simulink model "TTankModel"  (R2017b)
settings: Solver=FixedStepAuto  StartTime=62407  StopTime=120960  FixedStep=0.1  RelTol=1e-3
values from neighbouring files (symbols this model uses):
  intDelay = 20    [SingleFault.m]
  outTr = TTankModel_PCAtrainFunc(Xu_train)    [SingleFault.m]    (also in TTankModel_PCAtrainFunc.m = struct('mu_u',mu_u, 'sig_u',sigma_u,'PA', PA, 'LA', LA, 'A',)
  sizeStep_Gc11 = sensBias(1)    [SingleFault.m]    (also in faultCond.m = 0; steadyStateSet.m = 0)
  sizeStep_Gc23 = sensBias(2)    [SingleFault.m]    (also in faultCond.m = 0; steadyStateSet.m = 0)
  sizeStep_Gc32 = sensBias(3)    [SingleFault.m]    (also in faultCond.m = 0; steadyStateSet.m = 0)
  sizeStep_Gc44 = sensBias(4)    [SingleFault.m]    (also in faultCond.m = sensStep; steadyStateSet.m = 0)
  smDelay = 6    [SingleFault.m]
  tStep_Gc11 = sensTot(1,2)    [SingleFault.m]    (also in faultCond.m = 0; steadyStateSet.m = 0)
  tStep_Gc23 = sensTot(2,2)    [SingleFault.m]    (also in faultCond.m = 0; steadyStateSet.m = 0)
  tStep_Gc32 = sensTot(3,2)    [SingleFault.m]    (also in faultCond.m = 0; steadyStateSet.m = 0)
  tStep_Gc44 = sensTot(4,2)    [SingleFault.m]    (also in faultCond.m = sensTime; steadyStateSet.m = 0)
undefined symbols (not defined in the file or in its folder): ssOut
libraries: simulink x36
settings Model: Creator=17496594  LastModifiedBy=jtmccoy
settings DataIOCC: FinalStateName=SimStateTest  InitialState=stdyState  SaveCompleteFinalSimState=on  SaveFormat=Array  SignalLogging=off
settings CodeAppCC: StateflowObjectComments=on

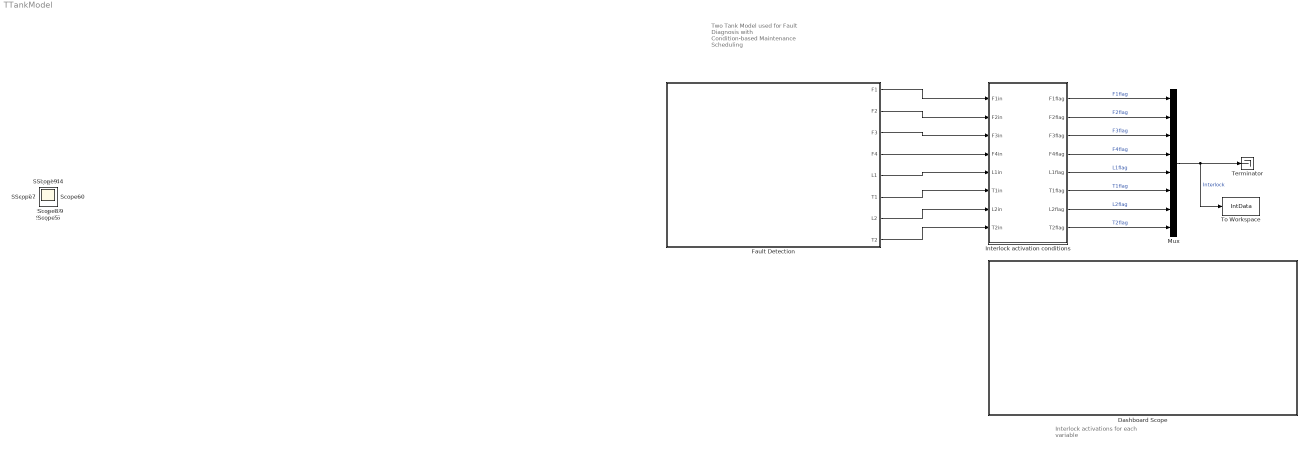
== system TTankModel ==
  note: Two Tank Model used for Fault Diagnosis
      | with Condition-based Maintenance Scheduling
  note: Interlock activations for each variable
  Dashboard Scope : Subsystem  DialogController=hmiCreateDDGDialog  IsWebBlock=on  mask(MWDashboardBlock){webBlockId=f2d3fcda-b4ff-4067-adce-a90dbe78b41d, webBlockType=sdiscope, ShowInitialText=on, HMISrcModelName=TTankModel}
      mask prompts: webBlockId "WebBlock Id"; webBlockType "WebBlock Type"; HMISrcModelName "Source Model"
      mask help: SimulinkHMI:dialogs:HMIScopeDialogDesc
      mask Help: helpview([docroot '/mapfiles/simulink.map'], 'hmi_scope')
      mask Display:
      | if strcmp(get_param(bdroot(gcb),'BlockDiagramType'), 'library')
      |     image([(matlabroot) '/toolbox/simulink/hmi/icons/DashboardScope.png']);
      | end
  Fault Detection : Subsystem
  Interlock activation conditions : Subsystem
  Mux : Mux  Inputs=8
  Terminator : Terminator
  To Workspace : ToWorkspace  VariableName=IntData  SampleTime=1
      settings: Save2DSignal=2-D array (concatenate along first dimension)
  Scope{,1..21} (22 alike) : Scope
  wires:
  Interlock activation conditions/2(F2flag) -> Mux/2  "F2flag"
  Fault Detection/8(T2) -> Interlock activation conditions/8(T2in)
  Fault Detection/7(L2) -> Interlock activation conditions/7(L2in)
  Fault Detection/5(L1) -> Interlock activation conditions/5(L1in)
  Fault Detection/6(T1) -> Interlock activation conditions/6(T1in)
  Fault Detection/4(F4) -> Interlock activation conditions/4(F4in)
  Fault Detection/3(F3) -> Interlock activation conditions/3(F3in)
  Fault Detection/2(F2) -> Interlock activation conditions/2("F2in ")
  Fault Detection/1(F1) -> Interlock activation conditions/1(F1in)
  Interlock activation conditions/8(T2flag) -> Mux/8  "T2flag"
  Mux/1 -> To Workspace/1, Terminator/1  "Interlock"
  Interlock activation conditions/7(L2flag) -> Mux/7  "L2flag"
  Interlock activation conditions/6(T1flag) -> Mux/6  "T1flag"
  Interlock activation conditions/5(L1flag) -> Mux/5  "L1flag"
  Interlock activation conditions/4(F4flag) -> Mux/4  "F4flag"
  Interlock activation conditions/1(F1flag) -> Mux/1  "F1flag"
  Interlock activation conditions/3(F3flag) -> Mux/3  "F3flag"

== system TTankModel/Dashboard Scope ==

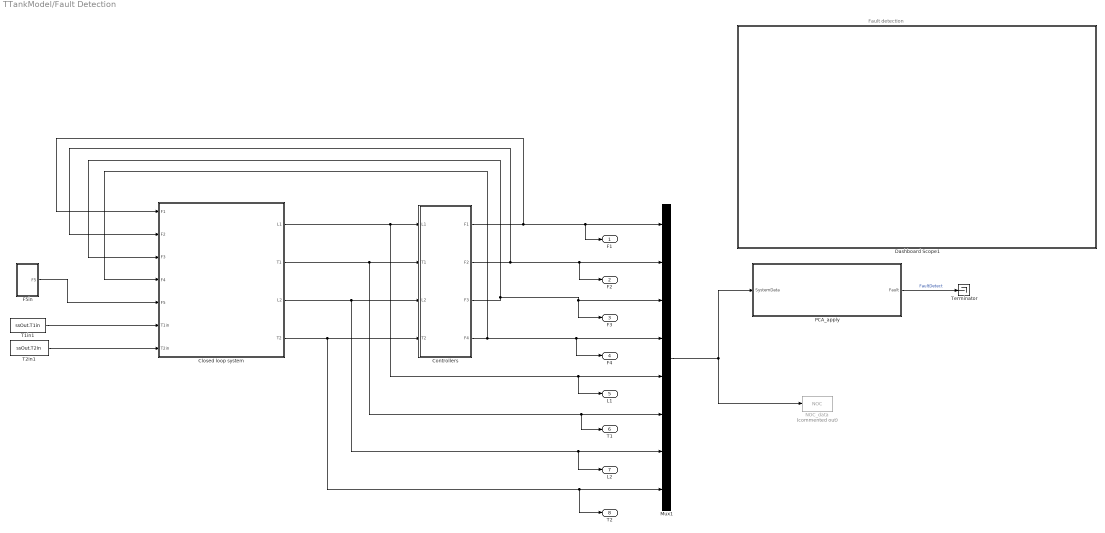
== system TTankModel/Fault Detection ==
  note: Fault detection
  Closed loop system : Subsystem
  Controllers : Subsystem
  Dashboard Scope1 : Subsystem  DialogController=hmiCreateDDGDialog  IsWebBlock=on  mask(MWDashboardBlock){webBlockId=01f67c63-4ebd-45d4-811d-95e04fe09010, webBlockType=sdiscope, ShowInitialText=on, HMISrcModelName=TTankModel}
      mask prompts: webBlockId "WebBlock Id"; webBlockType "WebBlock Type"; HMISrcModelName "Source Model"
      mask help: SimulinkHMI:dialogs:HMIScopeDialogDesc
      mask Help: helpview([docroot '/mapfiles/simulink.map'], 'hmi_scope')
      mask Display:
      | if strcmp(get_param(bdroot(gcb),'BlockDiagramType'), 'library')
      |     image([(matlabroot) '/toolbox/simulink/hmi/icons/DashboardScope.png']);
      | end
  F5in : Subsystem
  Mux1 : Mux  Inputs=8
  NOC_data : ToWorkspace  Commented=on  VariableName=NOC  SaveFormat=Timeseries  SampleTime=1
  PCA_apply : Subsystem
  T1in1 : Constant  Value=ssOut.T1in
  T2in1 : Constant  Value=ssOut.T2in
  Terminator : Terminator
  F1 : Outport
  F2 : Outport  Port=2
  F3 : Outport  Port=3
  F4 : Outport  Port=4
  L1 : Outport  Port=5
  T1 : Outport  Port=6
  L2 : Outport  Port=7
  T2 : Outport  Port=8
  wires:
  PCA_apply/1(Fault) -> Terminator/1  "FaultDetect"
  F5in/1(F5) -> Closed loop system/5(F5)
  Closed loop system/1(L1) -> Controllers/1(L1), L1/1, Mux1/5
  Mux1/1 -> PCA_apply/1(SystemData), NOC_data/1
  T1in1/1 -> Closed loop system/6(T1in)
  T2in1/1 -> Closed loop system/7(T2in)
  Closed loop system/4(T2) -> Controllers/4(T2), T2/1, Mux1/8
  Closed loop system/3(L2) -> Controllers/3(L2), L2/1, Mux1/7
  Closed loop system/2(T1) -> Controllers/2(T1), T1/1, Mux1/6
  Controllers/4(F4) -> Closed loop system/4(F4), F4/1, Mux1/4
  Controllers/2(F2) -> Closed loop system/2(F2), F2/1, Mux1/2
  Controllers/3(F3) -> Closed loop system/3(F3), F3/1, Mux1/3
  Controllers/1(F1) -> Closed loop system/1(F1), F1/1, Mux1/1

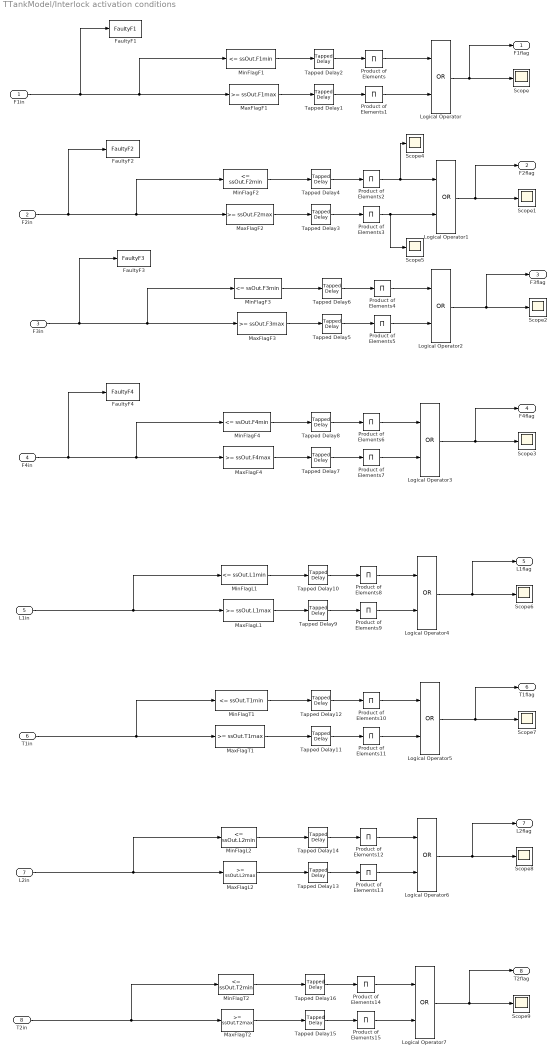
== system TTankModel/Interlock activation conditions ==
  F1in : Inport
  "F2in " : Inport  Port=2
  F3in : Inport  Port=3
  F4in : Inport  Port=4
  L1in : Inport  Port=5
  T1in : Inport  Port=6
  L2in : Inport  Port=7
  T2in : Inport  Port=8
  FaultyF1 : ToWorkspace  VariableName=FaultyF1  SaveFormat=Timeseries  SampleTime=-1
  FaultyF2 : ToWorkspace  VariableName=FaultyF2  SaveFormat=Timeseries  SampleTime=-1
  FaultyF3 : ToWorkspace  VariableName=FaultyF3  SaveFormat=Timeseries  SampleTime=-1
  FaultyF4 : ToWorkspace  VariableName=FaultyF4  SaveFormat=Timeseries  SampleTime=-1
  Logical Operator{,1..7} (8 alike) : Logic  Operator=OR  AllPortsSameDT=off  OutDataTypeStr=boolean
  MaxFlagF1 : simulink/Logic and Bit Operations/Compare To Constant  relop=>=  const=ssOut.F1max  OutDataTypeStr=boolean
  MaxFlagF2 : simulink/Logic and Bit Operations/Compare To Constant  relop=>=  const=ssOut.F2max  OutDataTypeStr=boolean
  MaxFlagF3 : simulink/Logic and Bit Operations/Compare To Constant  relop=>=  const=ssOut.F3max  OutDataTypeStr=boolean
  MaxFlagF4 : simulink/Logic and Bit Operations/Compare To Constant  relop=>=  const=ssOut.F4max  OutDataTypeStr=boolean
  MaxFlagL1 : simulink/Logic and Bit Operations/Compare To Constant  relop=>=  const=ssOut.L1max  OutDataTypeStr=boolean
  MaxFlagL2 : simulink/Logic and Bit Operations/Compare To Constant  relop=>=  const=ssOut.L2max  OutDataTypeStr=boolean
  MaxFlagT1 : simulink/Logic and Bit Operations/Compare To Constant  relop=>=  const=ssOut.T1max  OutDataTypeStr=boolean
  MaxFlagT2 : simulink/Logic and Bit Operations/Compare To Constant  relop=>=  const=ssOut.T2max  OutDataTypeStr=boolean
  MinFlagF1 : simulink/Logic and Bit Operations/Compare To Constant  relop=<=  const=ssOut.F1min  OutDataTypeStr=boolean
  MinFlagF2 : simulink/Logic and Bit Operations/Compare To Constant  relop=<=  const=ssOut.F2min  OutDataTypeStr=boolean
  MinFlagF3 : simulink/Logic and Bit Operations/Compare To Constant  relop=<=  const=ssOut.F3min  OutDataTypeStr=boolean
  MinFlagF4 : simulink/Logic and Bit Operations/Compare To Constant  relop=<=  const=ssOut.F4min  OutDataTypeStr=boolean
  MinFlagL1 : simulink/Logic and Bit Operations/Compare To Constant  relop=<=  const=ssOut.L1min  OutDataTypeStr=boolean
  MinFlagL2 : simulink/Logic and Bit Operations/Compare To Constant  relop=<=  const=ssOut.L2min  OutDataTypeStr=boolean
  MinFlagT1 : simulink/Logic and Bit Operations/Compare To Constant  relop=<=  const=ssOut.T1min  OutDataTypeStr=boolean
  MinFlagT2 : simulink/Logic and Bit Operations/Compare To Constant  relop=<=  const=ssOut.T2min  OutDataTypeStr=boolean
  Product of Elements{,1..15} (16 alike) : Product  Inputs=*
  Scope{,1..9} (10 alike) : Scope
  Tapped Delay{1..16} (16 alike) : simulink/Discrete/Tapped Delay  vinit=0.0  samptime=1  NumDelays=intDelay  DelayOrder=Oldest  includeCurrent=off
  F1flag : Outport
  F2flag : Outport  Port=2
  F3flag : Outport  Port=3
  F4flag : Outport  Port=4
  L1flag : Outport  Port=5
  T1flag : Outport  Port=6
  L2flag : Outport  Port=7
  T2flag : Outport  Port=8
  wires:
  MinFlagF1/1 -> Tapped Delay2/1
  MaxFlagF1/1 -> Tapped Delay1/1
  F1in/1 -> FaultyF1/1, MinFlagF1/1, MaxFlagF1/1
  Tapped Delay1/1 -> Product of Elements1/1
  Tapped Delay2/1 -> Product of Elements/1
  Product of Elements/1 -> Logical Operator/1
  Product of Elements1/1 -> Logical Operator/2
  Logical Operator/1 -> F1flag/1, Scope/1
  MinFlagF2/1 -> Tapped Delay4/1
  MaxFlagF2/1 -> Tapped Delay3/1
  "F2in "/1 -> MaxFlagF2/1, MinFlagF2/1, FaultyF2/1
  Tapped Delay3/1 -> Product of Elements3/1
  Tapped Delay4/1 -> Product of Elements2/1
  Product of Elements2/1 -> Scope4/1, Logical Operator1/1
  Product of Elements3/1 -> Scope5/1, Logical Operator1/2
  Logical Operator1/1 -> Scope1/1, F2flag/1
  MinFlagF3/1 -> Tapped Delay6/1
  MaxFlagF3/1 -> Tapped Delay5/1
  F3in/1 -> MaxFlagF3/1, MinFlagF3/1, FaultyF3/1
  Tapped Delay5/1 -> Product of Elements5/1
  Tapped Delay6/1 -> Product of Elements4/1
  Product of Elements4/1 -> Logical Operator2/1
  Product of Elements5/1 -> Logical Operator2/2
  Logical Operator2/1 -> Scope2/1, F3flag/1
  MinFlagF4/1 -> Tapped Delay8/1
  MaxFlagF4/1 -> Tapped Delay7/1
  F4in/1 -> MaxFlagF4/1, MinFlagF4/1, FaultyF4/1
  Tapped Delay7/1 -> Product of Elements7/1
  Tapped Delay8/1 -> Product of Elements6/1
  Product of Elements6/1 -> Logical Operator3/1
  Product of Elements7/1 -> Logical Operator3/2
  Logical Operator3/1 -> Scope3/1, F4flag/1
  MinFlagL1/1 -> Tapped Delay10/1
  MaxFlagL1/1 -> Tapped Delay9/1
  L1in/1 -> MaxFlagL1/1, MinFlagL1/1
  Tapped Delay9/1 -> Product of Elements9/1
  Tapped Delay10/1 -> Product of Elements8/1
  Product of Elements8/1 -> Logical Operator4/1
  Product of Elements9/1 -> Logical Operator4/2
  Logical Operator4/1 -> Scope6/1, L1flag/1
  MinFlagT1/1 -> Tapped Delay12/1
  MaxFlagT1/1 -> Tapped Delay11/1
  T1in/1 -> MaxFlagT1/1, MinFlagT1/1
  Tapped Delay11/1 -> Product of Elements11/1
  Tapped Delay12/1 -> Product of Elements10/1
  Product of Elements10/1 -> Logical Operator5/1
  Product of Elements11/1 -> Logical Operator5/2
  Logical Operator5/1 -> Scope7/1, T1flag/1
  MinFlagL2/1 -> Tapped Delay14/1
  MaxFlagL2/1 -> Tapped Delay13/1
  L2in/1 -> MaxFlagL2/1, MinFlagL2/1
  Tapped Delay13/1 -> Product of Elements13/1
  Tapped Delay14/1 -> Product of Elements12/1
  Product of Elements12/1 -> Logical Operator6/1
  Product of Elements13/1 -> Logical Operator6/2
  Logical Operator6/1 -> Scope8/1, L2flag/1
  MinFlagT2/1 -> Tapped Delay16/1
  MaxFlagT2/1 -> Tapped Delay15/1
  T2in/1 -> MaxFlagT2/1, MinFlagT2/1
  Tapped Delay15/1 -> Product of Elements15/1
  Tapped Delay16/1 -> Product of Elements14/1
  Product of Elements14/1 -> Logical Operator7/1
  Product of Elements15/1 -> Logical Operator7/2
  Logical Operator7/1 -> Scope9/1, T2flag/1

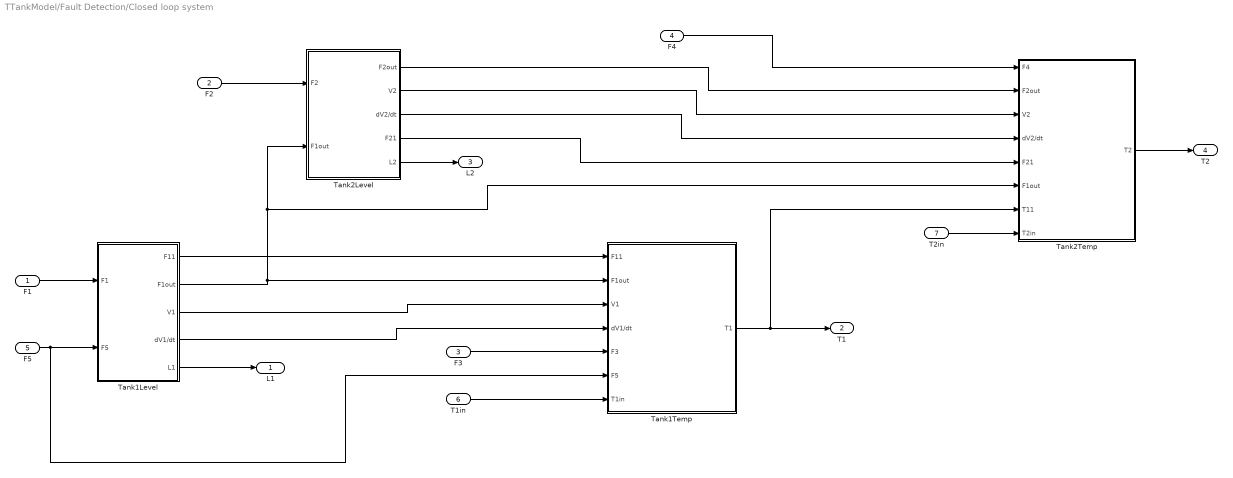
== system TTankModel/Fault Detection/Closed loop system ==
  F1 : Inport
  F2 : Inport  Port=2
  F3 : Inport  Port=3
  F4 : Inport  Port=4
  F5 : Inport  Port=5
  T1in : Inport  Port=6
  T2in : Inport  Port=7
  Tank1Level : Subsystem
  Tank1Temp : Subsystem
  Tank2Level : Subsystem
  Tank2Temp : Subsystem
  L1 : Outport
  T1 : Outport  Port=2
  L2 : Outport  Port=3
  T2 : Outport  Port=4
  wires:
  F1/1 -> Tank1Level/1(F1)
  Tank1Level/1(F11) -> Tank1Temp/1(F11)
  Tank1Temp/1(T1) -> Tank2Temp/7(T11), T1/1
  Tank1Level/3(V1) -> Tank1Temp/3(V1)
  Tank1Level/4(dV1/dt) -> Tank1Temp/4(dV1/dt)
  F3/1 -> Tank1Temp/5(F3)
  Tank1Level/2(F1out) -> Tank2Level/2(F1out), Tank2Temp/6(F1out), Tank1Temp/2(F1out)
  F2/1 -> Tank2Level/1(F2)
  Tank2Level/2(V2) -> Tank2Temp/3(V2)
  Tank2Level/1(F2out) -> Tank2Temp/2(F2out)
  Tank2Temp/1(T2) -> T2/1
  Tank2Level/3(dV2/dt) -> Tank2Temp/4(dV2/dt)
  Tank2Level/4(F21) -> Tank2Temp/5(F21)
  F4/1 -> Tank2Temp/1(F4)
  Tank1Level/5(L1) -> L1/1
  Tank2Level/5(L2) -> L2/1
  F5/1 -> Tank1Temp/6(F5), Tank1Level/2(F5)
  T1in/1 -> Tank1Temp/7(T1in)
  T2in/1 -> Tank2Temp/8(T2in)

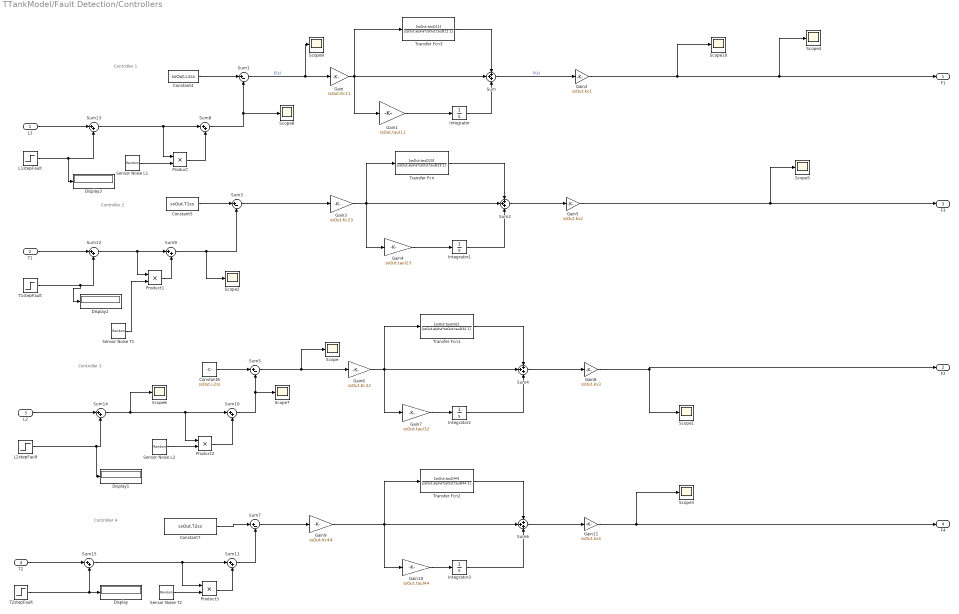
== system TTankModel/Fault Detection/Controllers ==
  note: Controller 1
  note: Controller 2
  note: Controller 3
  note: Controller 4
  L1 : Inport
  T1 : Inport  Port=2
  L2 : Inport  Port=3
  T2 : Inport  Port=4
  Constant4 : Constant  Value=ssOut.L1ss
  Constant5 : Constant  Value=ssOut.T1ss
  Constant6 : Constant  Value=ssOut.L2ss
  Constant7 : Constant  Value=ssOut.T2ss
  Display{,1..3} (4 alike) : Display
  Gain : Gain  Gain=ssOut.Kc11
  Gain1 : Gain  Gain=ssOut.tauI11
  Gain10 : Gain  Gain=ssOut.tauI44
  Gain11 : Gain  Gain=ssOut.kv4
  Gain2 : Gain  Gain=ssOut.kv1
  Gain3 : Gain  Gain=ssOut.Kc23
  Gain4 : Gain  Gain=ssOut.tauI23
  Gain5 : Gain  Gain=ssOut.kv2
  Gain6 : Gain  Gain=ssOut.Kc32
  Gain7 : Gain  Gain=ssOut.tauI32
  Gain8 : Gain  Gain=ssOut.kv3
  Gain9 : Gain  Gain=ssOut.Kc44
  Integrator : Integrator
  Integrator1 : Integrator  InitialCondition=ssOut.F3ss
  Integrator2 : Integrator  InitialCondition=ssOut.F2ss
  Integrator3 : Integrator  InitialCondition=ssOut.F4ss
  L1stepFault : Step  Time=tStep_Gc11  After=sizeStep_Gc11  SampleTime=0
  L2stepFault : Step  Time=tStep_Gc32  After=sizeStep_Gc32  SampleTime=0
  Product{,1..3} (4 alike) : Product
  Scope{,1..10} (11 alike) : Scope
  Sensor Noise L1 : UniformRandomNumber  Minimum=0  Maximum=ssOut.noiseL1  Seed=145  SampleTime=1
  Sensor Noise L2 : UniformRandomNumber  Minimum=0  Maximum=ssOut.noiseL2  Seed=145  SampleTime=1
  Sensor Noise T1 : UniformRandomNumber  Minimum=0  Maximum=ssOut.noiseT1  Seed=67  SampleTime=1
  Sensor Noise T2 : UniformRandomNumber  Minimum=0  Maximum=ssOut.noiseT2  Seed=67  SampleTime=1
  Sum{,2,4,6} (4 alike) : Sum  Inputs=+++
  Sum{1,3,5,7} (4 alike) : Sum  Inputs=|+-
  Sum{8..15} (8 alike) : Sum  Inputs=|++
  T1stepFault : Step  Time=tStep_Gc23  After=sizeStep_Gc23  SampleTime=0
  T2stepFault : Step  Time=tStep_Gc44  After=sizeStep_Gc44  SampleTime=0
  Transfer Fcn : TransferFcn  Numerator=[ssOut.tauD23]  Denominator=[ssOut.alpha*ssOut.tauD23 1]
  Transfer Fcn1 : TransferFcn  Numerator=[ssOut.tauD32]  Denominator=[ssOut.alpha*ssOut.tauD32 1]
  Transfer Fcn2 : TransferFcn  Numerator=[ssOut.tauD44]  Denominator=[ssOut.alpha*ssOut.tauD44 1]
  Transfer Fcn3 : TransferFcn  Numerator=[ssOut.tauD11]  Denominator=[ssOut.alpha*ssOut.tauD11 1]
  F1 : Outport
  F2 : Outport  Port=2
  F3 : Outport  Port=3
  F4 : Outport  Port=4
  wires:
  Transfer Fcn/1 -> Sum2/1
  Sum5/1 -> Scope/1, Gain6/1
  Transfer Fcn1/1 -> Sum4/1
  Sum4/1 -> Gain8/1
  Gain6/1 -> Transfer Fcn1/1, Gain7/1, Sum4/2
  Constant5/1 -> Sum3/1
  Sum3/1 -> Gain3/1
  Sum2/1 -> Gain5/1
  Gain7/1 -> Integrator2/1
  Integrator2/1 -> Sum4/3
  Constant6/1 -> Sum5/1
  Transfer Fcn2/1 -> Sum6/1
  Gain9/1 -> Transfer Fcn2/1, Gain10/1, Sum6/2
  Gain10/1 -> Integrator3/1
  Integrator3/1 -> Sum6/3
  Sum7/1 -> Gain9/1
  Constant7/1 -> Sum7/1
  Gain/1 -> Transfer Fcn3/1, Sum/2, Gain1/1
  Gain1/1 -> Integrator/1
  Integrator/1 -> Sum/3
  Sum1/1 -> Scope9/1, Gain/1  "E(s)"
  Sum/1 -> Gain2/1  "P(s)"
  Constant4/1 -> Sum1/1
  Sum6/1 -> Gain11/1
  Integrator1/1 -> Sum2/3
  Gain4/1 -> Integrator1/1
  Gain3/1 -> Transfer Fcn/1, Gain4/1, Sum2/2
  Transfer Fcn3/1 -> Sum/1
  Product/1 -> Sum8/2
  Sensor Noise L1/1 -> Product/2
  Sum8/1 -> Scope8/1, Sum1/2
  Sum9/1 -> Scope2/1, Sum3/2
  Product1/1 -> Sum9/2
  Sensor Noise T1/1 -> Product1/2
  Sum10/1 -> Scope7/1, Sum5/2
  Product2/1 -> Sum10/2
  Sensor Noise L2/1 -> Product2/2
  Sum11/1 -> Sum7/2
  Product3/1 -> Sum11/2
  Sensor Noise T2/1 -> Product3/2
  T1/1 -> Sum12/1
  Sum12/1 -> Product1/1, Sum9/1
  T1stepFault/1 -> Display2/1, Sum12/2
  L1/1 -> Sum13/1
  Sum13/1 -> Product/1, Sum8/1
  L1stepFault/1 -> Display3/1, Sum13/2
  T2/1 -> Sum15/1
  Sum15/1 -> Product3/1, Sum11/1
  T2stepFault/1 -> Display/1, Sum15/2
  L2/1 -> Sum14/1
  Sum14/1 -> Scope6/1, Product2/1, Sum10/1
  L2stepFault/1 -> Display1/1, Sum14/2
  Gain2/1 -> Scope10/1, F1/1, Scope4/1
  Gain5/1 -> F3/1, Scope5/1
  Gain8/1 -> F2/1, Scope1/1
  Gain11/1 -> F4/1, Scope3/1

== system TTankModel/Fault Detection/Dashboard Scope1 ==

== system TTankModel/Fault Detection/F5in ==
  Constant : Constant  Value=ssOut.F5ss
  F5 RW : Subsystem
  Product : Product
  Scope : Scope
  Sum : Sum  Inputs=++|
  To Workspace : ToWorkspace  VariableName=F5out  SampleTime=-1
      settings: Save2DSignal=2-D array (concatenate along first dimension)
  F5 : Outport
  wires:
  Sum/1 -> Scope/1, To Workspace/1, F5/1
  Product/1 -> Sum/1
  Constant/1 -> Product/1, Sum/2
  F5 RW/1(y) -> Product/2

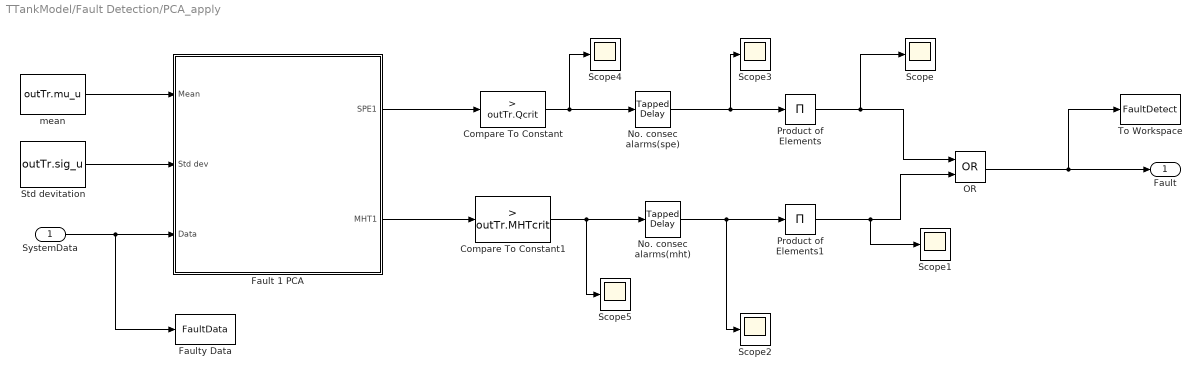
== system TTankModel/Fault Detection/PCA_apply ==
  SystemData : Inport
  Compare To Constant : simulink/Logic and Bit Operations/Compare To Constant  relop=>  const=outTr.Qcrit  OutDataTypeStr=boolean
  Compare To Constant1 : simulink/Logic and Bit Operations/Compare To Constant  relop=>  const=outTr.MHTcrit  OutDataTypeStr=boolean
  Fault 1 PCA : Subsystem
  Faulty Data : ToWorkspace  VariableName=FaultData  SampleTime=1
      settings: Save2DSignal=2-D array (concatenate along first dimension)
  No. consec alarms(mht) : simulink/Discrete/Tapped Delay  vinit=0.0  samptime=1  NumDelays=smDelay  DelayOrder=Oldest  includeCurrent=off
  No. consec alarms(spe) : simulink/Discrete/Tapped Delay  vinit=0.0  samptime=1  NumDelays=smDelay  DelayOrder=Oldest  includeCurrent=off
  OR : Logic  Operator=OR  AllPortsSameDT=off  OutDataTypeStr=boolean
  Product of Elements : Product  Inputs=*  CollapseDim=2
  Product of Elements1 : Product  Inputs=*
  Scope{,1..5} (6 alike) : Scope
  Std devitation : Constant  Value=outTr.sig_u
  To Workspace : ToWorkspace  VariableName=FaultDetect  SampleTime=1
      settings: Save2DSignal=2-D array (concatenate along first dimension)
  mean : Constant  Value=outTr.mu_u
  Fault : Outport
  wires:
  Fault 1 PCA/1(SPE1) -> Compare To Constant/1
  Std devitation/1 -> Fault 1 PCA/2(Std dev)
  mean/1 -> Fault 1 PCA/1(Mean)
  Fault 1 PCA/2(MHT1) -> Compare To Constant1/1
  SystemData/1 -> Faulty Data/1, Fault 1 PCA/3(Data)
  Compare To Constant1/1 -> Scope5/1, No. consec alarms(mht)/1
  No. consec alarms(spe)/1 -> Scope3/1, Product of Elements/1
  OR/1 -> Fault/1, To Workspace/1
  Product of Elements/1 -> Scope/1, OR/1
  Product of Elements1/1 -> Scope1/1, OR/2
  No. consec alarms(mht)/1 -> Scope2/1, Product of Elements1/1
  Compare To Constant/1 -> Scope4/1, No. consec alarms(spe)/1

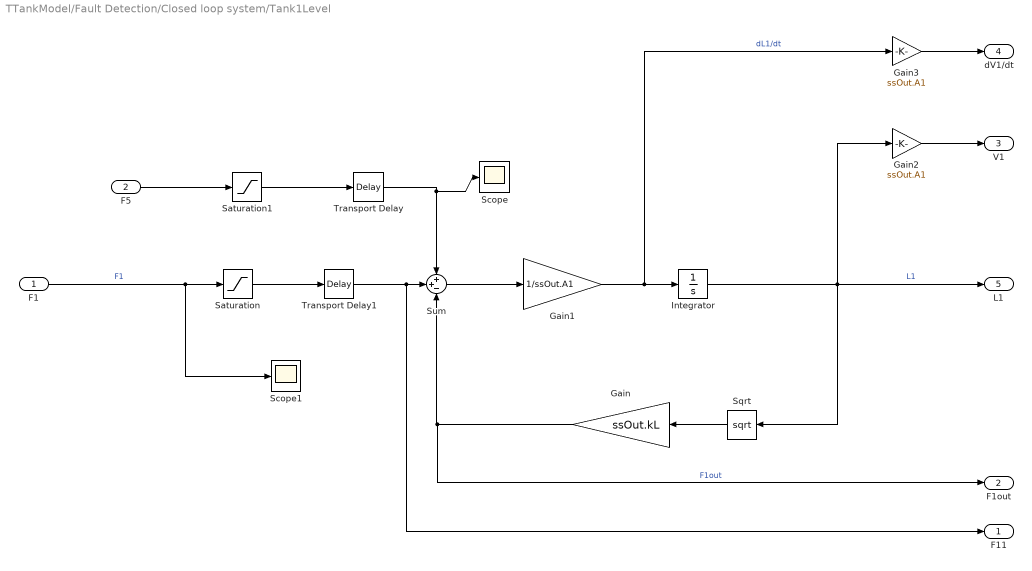
== system TTankModel/Fault Detection/Closed loop system/Tank1Level ==
  F1 : Inport
  F5 : Inport  Port=2
  Gain : Gain  Gain=ssOut.kL
  Gain1 : Gain  Gain=1/ssOut.A1
  Gain2 : Gain  Gain=ssOut.A1
  Gain3 : Gain  Gain=ssOut.A1
  Integrator : Integrator  InitialCondition=ssOut.L1ss
  Saturation : Saturate  UpperLimit=ssOut.F1max  LowerLimit=ssOut.F1min
  Saturation1 : Saturate  UpperLimit=0.2  LowerLimit=0
  Scope : Scope
  Scope1 : Scope
  Sqrt : Sqrt  SaturateOnIntegerOverflow=on
  Sum : Sum  Inputs=++-
  Transport Delay : TransportDelay  DelayTime=1.2
  Transport Delay1 : TransportDelay  DelayTime=1.2
  F11 : Outport
  F1out : Outport  Port=2
  V1 : Outport  Port=3
  dV1/dt : Outport  Port=4
  L1 : Outport  Port=5
  wires:
  Gain/1 -> Sum/3, F1out/1  "F1out"
  F1/1 -> Scope1/1, Saturation/1  "F1"
  Sqrt/1 -> Gain/1
  Sum/1 -> Gain1/1
  Integrator/1 -> Gain2/1, L1/1, Sqrt/1  "L1"
  Gain1/1 -> Gain3/1, Integrator/1  "dL1/dt"
  Gain2/1 -> V1/1
  Gain3/1 -> dV1/dt/1
  F5/1 -> Saturation1/1
  Saturation1/1 -> Transport Delay/1
  Transport Delay/1 -> Scope/1, Sum/1
  Transport Delay1/1 -> Sum/2, F11/1
  Saturation/1 -> Transport Delay1/1

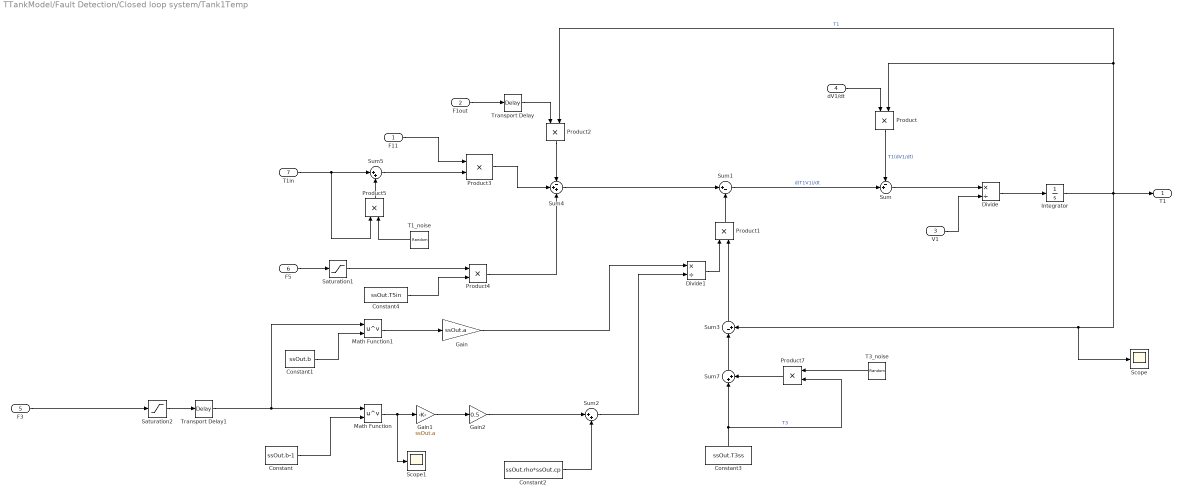
== system TTankModel/Fault Detection/Closed loop system/Tank1Temp ==
  F11 : Inport
  F1out : Inport  Port=2
  V1 : Inport  Port=3
  dV1/dt : Inport  Port=4
  F3 : Inport  Port=5
  F5 : Inport  Port=6
  T1in : Inport  Port=7
  Constant : Constant  Value=ssOut.b-1
  Constant1 : Constant  Value=ssOut.b
  Constant2 : Constant  Value=ssOut.rho*ssOut.cp
  Constant3 : Constant  Value=ssOut.T3ss
  Constant4 : Constant  Value=ssOut.T5in
  Divide : Product  Inputs=*/
  Divide1 : Product  Inputs=*/
  Gain : Gain  Gain=ssOut.a
  Gain1 : Gain  Gain=ssOut.a
  Gain2 : Gain  Gain=0.5
  Integrator : Integrator  InitialCondition=ssOut.T1ss
  Math Function : Math  Operator=pow  SaturateOnIntegerOverflow=on
  Math Function1 : Math  Operator=pow  SaturateOnIntegerOverflow=on
  Product{,1..5,7} (7 alike) : Product
  Saturation1 : Saturate  UpperLimit=0.2  LowerLimit=0
  Saturation2 : Saturate  UpperLimit=ssOut.F3max  LowerLimit=ssOut.F3min
  Scope : Scope
  Scope1 : Scope
  Sum : Sum  Inputs=-+|
  Sum1 : Sum  Inputs=|+-
  Sum2 : Sum  Inputs=|++
  Sum3 : Sum  Inputs=|-+
  Sum4 : Sum  Inputs=-++
  Sum5 : Sum  Inputs=|++
  Sum7 : Sum  Inputs=|++
  T1_noise : RandomNumber  Variance=ssOut.noiseT1in  Seed=20  SampleTime=1
  T3_noise : RandomNumber  Variance=ssOut.noiseT3  Seed=22  SampleTime=1
  Transport Delay : TransportDelay  DelayTime=0.8
  Transport Delay1 : TransportDelay  DelayTime=1.2
  T1 : Outport
  wires:
  dV1/dt/1 -> Product/1
  Sum2/1 -> Divide1/2
  Constant1/1 -> Math Function1/2
  Sum1/1 -> Sum/2  "d(T1V1)/dt"
  Integrator/1 -> T1/1, Scope/1, Sum3/2, Product2/2, Product/2  "T1"
  Divide/1 -> Integrator/1
  Math Function1/1 -> Gain/1
  V1/1 -> Divide/2
  Constant/1 -> Math Function/2
  Product/1 -> Sum/1  "T1(dV1/dt)"
  Constant2/1 -> Sum2/2
  Gain/1 -> Divide1/1
  Sum/1 -> Divide/1
  Sum3/1 -> Product1/2
  Product1/1 -> Sum1/2
  Divide1/1 -> Product1/1
  Gain2/1 -> Sum2/1
  Math Function/1 -> Scope1/1, Gain1/1
  Gain1/1 -> Gain2/1
  Constant3/1 -> Product7/2, Sum7/1  "T3"
  Product2/1 -> Sum4/1
  Sum4/1 -> Sum1/1
  F11/1 -> Product3/1
  F1out/1 -> Transport Delay/1
  Product3/1 -> Sum4/2
  T1in/1 -> Product5/1, Sum5/1
  F5/1 -> Saturation1/1
  Constant4/1 -> Product4/2
  Product4/1 -> Sum4/3
  F3/1 -> Saturation2/1
  Saturation1/1 -> Product4/1
  Transport Delay/1 -> Product2/1
  Sum5/1 -> Product3/2
  Product5/1 -> Sum5/2
  T1_noise/1 -> Product5/2
  Transport Delay1/1 -> Math Function1/1, Math Function/1
  Product7/1 -> Sum7/2
  T3_noise/1 -> Product7/1
  Sum7/1 -> Sum3/1
  Saturation2/1 -> Transport Delay1/1

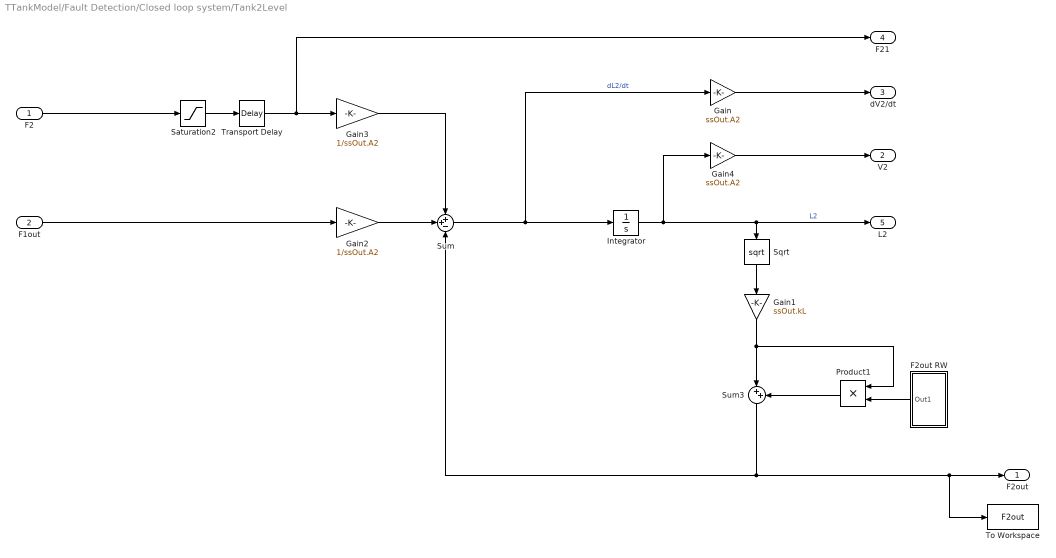
== system TTankModel/Fault Detection/Closed loop system/Tank2Level ==
  F2 : Inport
  F1out : Inport  Port=2
  F2out RW : Subsystem
  Gain : Gain  Gain=ssOut.A2
  Gain1 : Gain  Gain=ssOut.kL
  Gain2 : Gain  Gain=1/ssOut.A2
  Gain3 : Gain  Gain=1/ssOut.A2
  Gain4 : Gain  Gain=ssOut.A2
  Integrator : Integrator  InitialCondition=ssOut.L2ss
  Product1 : Product
  Saturation2 : Saturate  UpperLimit=ssOut.F2max  LowerLimit=0
  Sqrt : Sqrt  SaturateOnIntegerOverflow=on
  Sum : Sum  Inputs=++-
  Sum3 : Sum  Inputs=|++
  To Workspace : ToWorkspace  VariableName=F2out  SaveFormat=Timeseries  SampleTime=1
  Transport Delay : TransportDelay  DelayTime=1.2
  F2out : Outport
  V2 : Outport  Port=2
  dV2/dt : Outport  Port=3
  F21 : Outport  Port=4
  L2 : Outport  Port=5
  wires:
  Integrator/1 -> Gain4/1, L2/1, Sqrt/1  "L2"
  Sum/1 -> Gain/1, Integrator/1  "dL2/dt"
  Sqrt/1 -> Gain1/1
  F1out/1 -> Gain2/1
  Gain2/1 -> Sum/2
  Gain3/1 -> Sum/1
  Gain4/1 -> V2/1
  Gain/1 -> dV2/dt/1
  Saturation2/1 -> Transport Delay/1
  F2/1 -> Saturation2/1
  Transport Delay/1 -> F21/1, Gain3/1
  Gain1/1 -> Product1/1, Sum3/1
  Sum3/1 -> To Workspace/1, F2out/1, Sum/3
  Product1/1 -> Sum3/2
  F2out RW/1(Out1) -> Product1/2

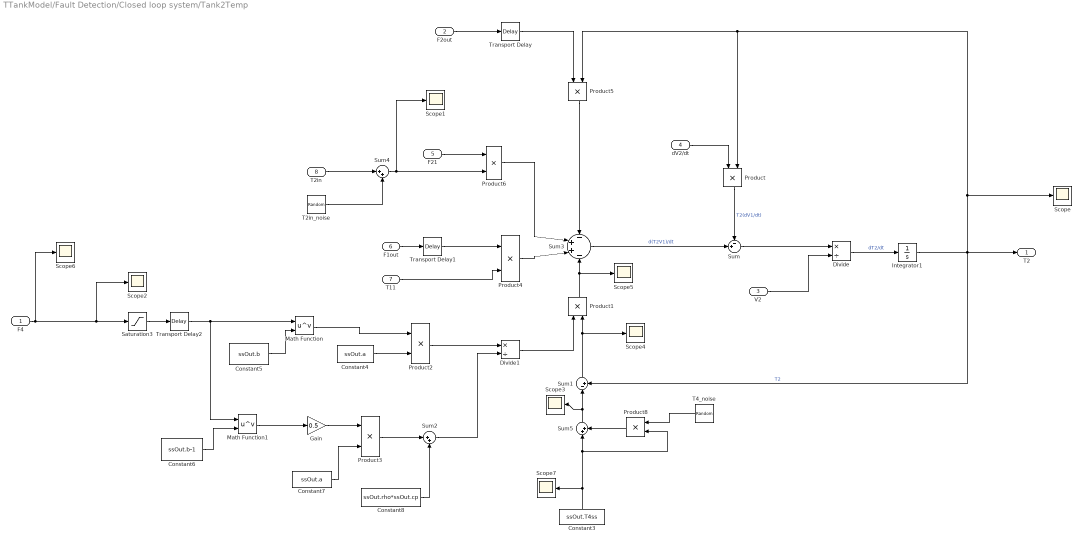
== system TTankModel/Fault Detection/Closed loop system/Tank2Temp ==
  F4 : Inport
  F2out : Inport  Port=2
  V2 : Inport  Port=3
  dV2/dt : Inport  Port=4
  F21 : Inport  Port=5
  F1out : Inport  Port=6
  T11 : Inport  Port=7
  T2in : Inport  Port=8
  Constant3 : Constant  Value=ssOut.T4ss
  Constant4 : Constant  Value=ssOut.a
  Constant5 : Constant  Value=ssOut.b
  Constant6 : Constant  Value=ssOut.b-1
  Constant7 : Constant  Value=ssOut.a
  Constant8 : Constant  Value=ssOut.rho*ssOut.cp
  Divide : Product  Inputs=*/
  Divide1 : Product  Inputs=*/
  Gain : Gain  Gain=0.5
  Integrator1 : Integrator  InitialCondition=ssOut.T2ss
  Math Function : Math  Operator=pow  SaturateOnIntegerOverflow=on
  Math Function1 : Math  Operator=pow  SaturateOnIntegerOverflow=on
  Product{,1..6,8} (8 alike) : Product
  Saturation3 : Saturate  UpperLimit=ssOut.F4max  LowerLimit=0
  Scope{,1..7} (8 alike) : Scope
  Sum : Sum  Inputs=-+|
  Sum1 : Sum  Inputs=|-+
  Sum2 : Sum  Inputs=|++
  Sum3 : Sum  Inputs=-++-
  Sum4 : Sum  Inputs=|++
  Sum5 : Sum  Inputs=|++
  T2in_noise : RandomNumber  Variance=ssOut.noiseT2in  Seed=25  SampleTime=1
  T4_noise : RandomNumber  Variance=ssOut.noiseT4  Seed=84  SampleTime=1
  Transport Delay : TransportDelay  DelayTime=1.2
  Transport Delay1 : TransportDelay  DelayTime=1.2
  Transport Delay2 : TransportDelay  DelayTime=1.2
  T2 : Outport
  wires:
  Math Function1/1 -> Gain/1
  Sum2/1 -> Divide1/2
  Math Function/1 -> Product2/1
  Divide1/1 -> Product1/1
  Product5/1 -> Sum3/1
  F2out/1 -> Transport Delay/1
  Product3/1 -> Sum2/1
  Gain/1 -> Product3/1
  Constant7/1 -> Product3/2
  F1out/1 -> Transport Delay1/1
  Constant4/1 -> Product2/2
  Constant5/1 -> Math Function/2
  T2in/1 -> Sum4/1
  T11/1 -> Product4/2
  Product6/1 -> Sum3/2
  F21/1 -> Product6/1
  Constant8/1 -> Sum2/2
  Product4/1 -> Sum3/3
  Sum1/1 -> Scope4/1, Product1/2
  Product1/1 -> Scope5/1, Sum3/4
  Product2/1 -> Divide1/1
  dV2/dt/1 -> Product/1
  V2/1 -> Divide/2
  Product/1 -> Sum/1  "T2(dV1/dt)"
  Integrator1/1 -> T2/1, Sum1/2, Scope/1, Product5/2, Product/2  "T2"
  Sum3/1 -> Sum/2  "d(T2V1)/dt"
  Sum/1 -> Divide/1
  Divide/1 -> Integrator1/1  "dT2/dt"
  Constant6/1 -> Math Function1/2
  F4/1 -> Saturation3/1, Scope2/1, Scope6/1
  Transport Delay/1 -> Product5/1
  Sum4/1 -> Scope1/1, Product6/2
  Transport Delay1/1 -> Product4/1
  Sum5/1 -> Scope3/1, Sum1/1
  Product8/1 -> Sum5/2
  T4_noise/1 -> Product8/1
  Transport Delay2/1 -> Math Function1/1, Math Function/1
  T2in_noise/1 -> Sum4/2
  Constant3/1 -> Scope7/1, Product8/2, Sum5/1
  Saturation3/1 -> Transport Delay2/1

== system TTankModel/Fault Detection/F5in/F5 RW ==
  note: reduce amplitube by dividng by a constant
  Constant2 : Constant  Value=10
  Delay : Delay  DelayLength=1
  Divide : Product  Inputs=*/
  Gain : Gain  Gain=0.08
  Random Number : RandomNumber  Variance=0.0019  Seed=5  SampleTime=1
  Scope1 : Scope
  Sum : Sum  Inputs=|++
  y : Outport
  wires:
  Delay/1 -> Gain/1
  Gain/1 -> Sum/1
  Random Number/1 -> Sum/2
  Sum/1 -> Divide/1
  Constant2/1 -> Divide/2
  Divide/1 -> y/1, Scope1/1, Delay/1

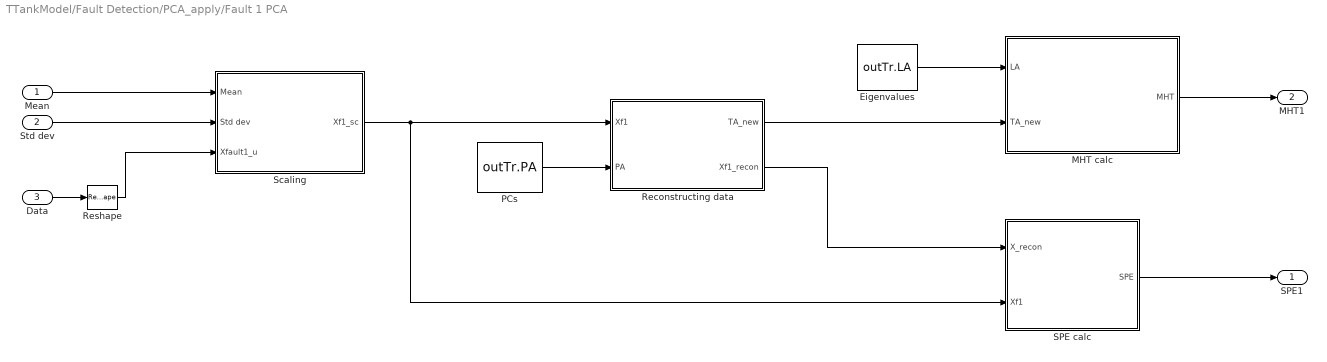
== system TTankModel/Fault Detection/PCA_apply/Fault 1 PCA ==
  Mean : Inport
  Std dev : Inport  Port=2
  Data : Inport  Port=3
  Eigenvalues : Constant  Value=outTr.LA
  MHT calc : Subsystem
  PCs : Constant  Value=outTr.PA
  Reconstructing data : Subsystem
  Reshape : Reshape  OutputDimensionality=Row vector (2-D)
  SPE calc : Subsystem
  Scaling : Subsystem
  SPE1 : Outport
  MHT1 : Outport  Port=2
  wires:
  Mean/1 -> Scaling/1(Mean)
  Std dev/1 -> Scaling/2(Std dev)
  Scaling/1(Xf1_sc) -> SPE calc/2(Xf1), Reconstructing data/1(Xf1)
  PCs/1 -> Reconstructing data/2(PA)
  Reconstructing data/1(TA_new) -> MHT calc/2(TA_new)
  Eigenvalues/1 -> MHT calc/1(LA)
  Reconstructing data/2(Xf1_recon) -> SPE calc/1(X_recon)
  MHT calc/1(MHT) -> MHT1/1
  Data/1 -> Reshape/1
  Reshape/1 -> Scaling/3(Xfault1_u)
  SPE calc/1(SPE) -> SPE1/1

== system TTankModel/Fault Detection/Closed loop system/Tank2Level/F2out RW ==
  Constant2 : Constant  Value=3
  Delay : Delay  DelayLength=1
  Divide : Product  Inputs=*/
  Gain : Gain  Gain=0.08
  Random Number : RandomNumber  Variance=0.019  Seed=80  SampleTime=1
  Scope1 : Scope
  Sum : Sum  Inputs=|++
  Out1 : Outport
  wires:
  Delay/1 -> Gain/1
  Gain/1 -> Sum/1
  Random Number/1 -> Sum/2
  Sum/1 -> Divide/1
  Constant2/1 -> Divide/2
  Divide/1 -> Out1/1, Scope1/1, Delay/1

== system TTankModel/Fault Detection/PCA_apply/Fault 1 PCA/MHT calc ==
  LA : Inport
  TA_new : Inport  Port=2
  Divide : Product  Inputs=*/
  Matrix Sum : Sum  Inputs=+  CollapseMode=Specified dimension  CollapseDim=2
  Square : Math  Operator=square  SaturateOnIntegerOverflow=on
  To Workspace : ToWorkspace  VariableName=MHTtotal  SampleTime=1
      settings: Save2DSignal=2-D array (concatenate along first dimension)
  To Workspace1 : ToWorkspace  VariableName=MHTall  SampleTime=1
      settings: Save2DSignal=2-D array (concatenate along first dimension)
  Transpose : Math  Operator=transpose  SaturateOnIntegerOverflow=on
  MHT : Outport
  wires:
  Transpose/1 -> Divide/2
  Square/1 -> Divide/1
  TA_new/1 -> Square/1
  Matrix Sum/1 -> To Workspace/1, MHT/1  "MHT"
  LA/1 -> Transpose/1
  Divide/1 -> To Workspace1/1, Matrix Sum/1

== system TTankModel/Fault Detection/PCA_apply/Fault 1 PCA/Reconstructing data ==
  Xf1 : Inport
  PA : Inport  Port=2
  Math Function : Math  Operator=transpose  SaturateOnIntegerOverflow=on
  Matrix Multiply : Product  Multiplication=Matrix(*)
  Product : Product  Inputs=**  Multiplication=Matrix(*)  OutDataTypeStr=Inherit: Same as first input
  TA_new : Outport
  Xf1_recon : Outport  Port=2
  wires:
  Math Function/1 -> Matrix Multiply/2
  PA/1 -> Math Function/1, Product/2
  Xf1/1 -> Product/1
  Matrix Multiply/1 -> Xf1_recon/1  "Xf1_recon"
  Product/1 -> Matrix Multiply/1, TA_new/1  "TA_new"

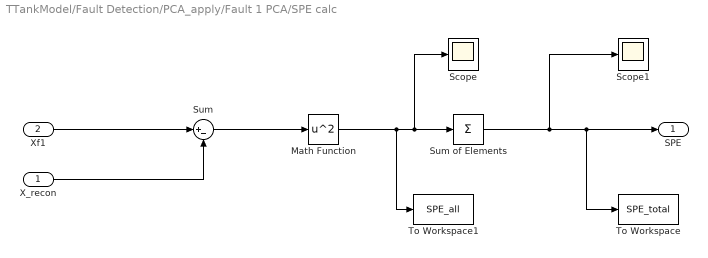
== system TTankModel/Fault Detection/PCA_apply/Fault 1 PCA/SPE calc ==
  X_recon : Inport
  Xf1 : Inport  Port=2
  Math Function : Math  Operator=square
  Scope : Scope
  Scope1 : Scope
  Sum : Sum  Inputs=|+-
  Sum of Elements : Sum  Inputs=+  CollapseMode=Specified dimension  CollapseDim=2
  To Workspace : ToWorkspace  VariableName=SPE_total  SampleTime=1
      settings: Save2DSignal=2-D array (concatenate along first dimension)
  To Workspace1 : ToWorkspace  VariableName=SPE_all  SampleTime=1
      settings: Save2DSignal=2-D array (concatenate along first dimension)
  SPE : Outport
  wires:
  Sum of Elements/1 -> Scope1/1, To Workspace/1, SPE/1
  Sum/1 -> Math Function/1
  Math Function/1 -> To Workspace1/1, Scope/1, Sum of Elements/1
  Xf1/1 -> Sum/1
  X_recon/1 -> Sum/2

== system TTankModel/Fault Detection/PCA_apply/Fault 1 PCA/Scaling ==
  Mean : Inport
  Std dev : Inport  Port=2
  Xfault1_u : Inport  Port=3
  Divide : Product  Inputs=*/  OutDataTypeStr=Inherit: Same as first input
  Sum : Sum  Inputs=|+-  OutDataTypeStr=Inherit: Same as first input
  Xf1_sc : Outport
  wires:
  Std dev/1 -> Divide/2
  Divide/1 -> Xf1_sc/1
  Xfault1_u/1 -> Sum/1
  Mean/1 -> Sum/2
  Sum/1 -> Divide/1
